simulink model "mytestmdl"  (Simulink 7.8)
settings: Solver=ode45  StartTime=0.0  StopTime=1  MaxStep=2e-5  RelTol=1e-3
values from neighbouring files (symbols this model uses):
  b = 1    [sim_parallel.m]    (also in sim_serial.m)
  k = 1;'])    [sim_parallel.m]    (also in sim_serial.m = 1)
settings Model: Creator=tmuppira  LastModifiedBy=tmuppira

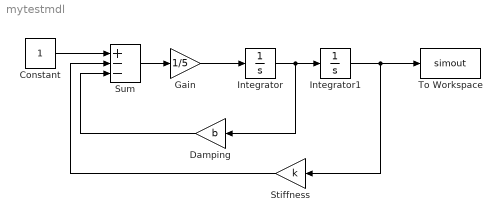
== system mytestmdl ==
  Constant : Constant
  Damping : Gain  Gain=b
  Gain : Gain  Gain=1/5
  Integrator : Integrator
  Integrator1 : Integrator
  Stiffness : Gain  Gain=k
  Sum : Sum  Inputs=+--
  To Workspace : ToWorkspace  VariableName=simout  SampleTime=1e-2  SaveFormat=Array
  wires:
  Integrator1/1 -> To Workspace/1, Stiffness/1
  Integrator/1 -> Integrator1/1, Damping/1
  Gain/1 -> Integrator/1
  Stiffness/1 -> Sum/2
  Sum/1 -> Gain/1
  Constant/1 -> Sum/1
  Damping/1 -> Sum/3
